simulink library "Rotation"  (R2018b)
settings: Solver=VariableStepAuto  StartTime=0.0  StopTime=10.0  RelTol=1e-3
settings Model: Creator=zouji  LastModifiedBy=zouji

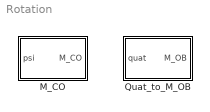
== system Rotation ==
  M_CO : Subsystem
  Quat_to_M_OB : Subsystem

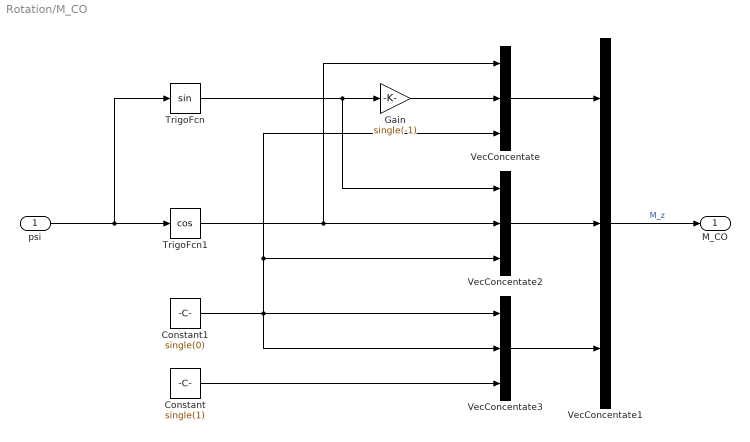
== system Rotation/M_CO ==
  psi : Inport  Unit=rad  PortDimensions=1
      settings: AttributesFormatString=Unit: %<Unit>
  Constant : Constant  Value=single(1)  VectorParams1D=off  OutDataTypeStr=Inherit: Inherit via back propagation
      settings: AttributesFormatString=Value: %<Value>
  Constant1 : Constant  Value=single(0)  VectorParams1D=off  OutDataTypeStr=Inherit: Inherit via back propagation
      settings: AttributesFormatString=Value: %<Value>
  Gain : Gain  Gain=single(-1)  OutDataTypeStr=Inherit: Same as input  ParamDataTypeStr=Inherit: Same as input
      settings: AttributesFormatString=Gain: %<Gain>
  TrigoFcn : Trigonometry  OutputSignalType=real
  TrigoFcn1 : Trigonometry  Operator=cos  OutputSignalType=real
  VecConcentate : Concatenate  NumInputs=3  Mode=Multidimensional array
  VecConcentate1 : Concatenate  NumInputs=3  Mode=Multidimensional array  ConcatenateDimension=2
  VecConcentate2 : Concatenate  NumInputs=3  Mode=Multidimensional array
  VecConcentate3 : Concatenate  NumInputs=3  Mode=Multidimensional array
  M_CO : Outport  Unit=1  PortDimensions=[3,3]
      settings: AttributesFormatString=Unit: %<Unit>
  wires:
  Constant1/1 -> VecConcentate/3, VecConcentate2/3, VecConcentate3/2, VecConcentate3/1
  TrigoFcn1/1 -> VecConcentate/1, VecConcentate2/2
  psi/1 -> TrigoFcn/1, TrigoFcn1/1
  VecConcentate1/1 -> M_CO/1  "M_z"
  VecConcentate/1 -> VecConcentate1/1
  VecConcentate2/1 -> VecConcentate1/2
  VecConcentate3/1 -> VecConcentate1/3
  TrigoFcn/1 -> VecConcentate2/1, Gain/1
  Gain/1 -> VecConcentate/2
  Constant/1 -> VecConcentate3/3

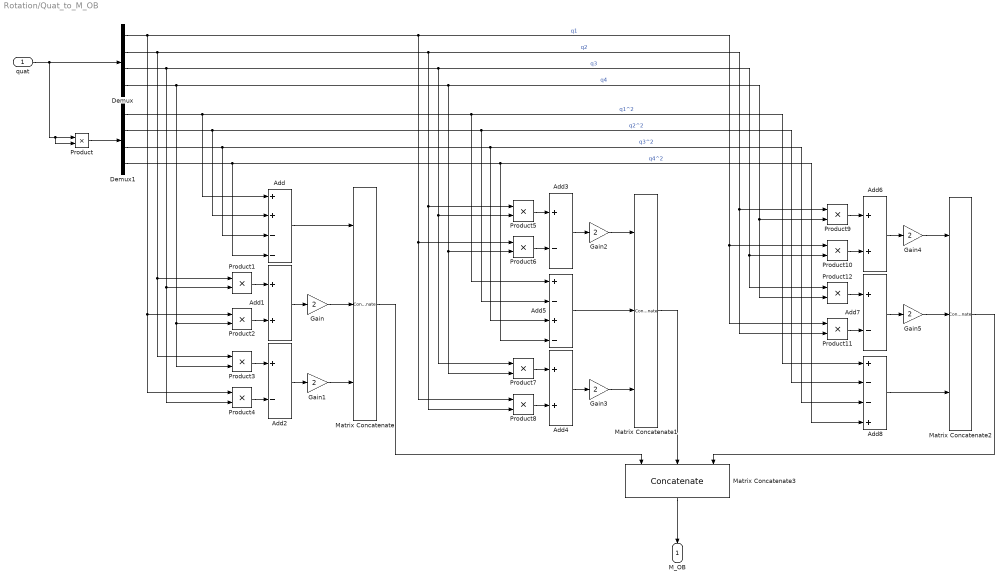
== system Rotation/Quat_to_M_OB ==
  quat : Inport
  Add : Sum  Inputs=++--
  Add1 : Sum
  Add2 : Sum  Inputs=+-
  Add3 : Sum  Inputs=+-
  Add4 : Sum
  Add5 : Sum  Inputs=+-+-
  Add6 : Sum
  Add7 : Sum  Inputs=+-
  Add8 : Sum  Inputs=+--+
  Demux : Demux
  Demux1 : Demux
  Gain{,1..5} (6 alike) : Gain  Gain=2  OutDataTypeStr=Inherit: Same as input
  Matrix Concatenate : Concatenate  NumInputs=3
  Matrix Concatenate1 : Concatenate  NumInputs=3
  Matrix Concatenate2 : Concatenate  NumInputs=3
  Matrix Concatenate3 : Concatenate  NumInputs=3  Mode=Multidimensional array  ConcatenateDimension=2
  Product{,1..12} (13 alike) : Product  RndMeth=Zero
  M_OB : Outport
  wires:
  Matrix Concatenate3/1 -> M_OB/1
  Matrix Concatenate2/1 -> Matrix Concatenate3/3
  Matrix Concatenate1/1 -> Matrix Concatenate3/2
  Matrix Concatenate/1 -> Matrix Concatenate3/1
  Add8/1 -> Matrix Concatenate2/3
  Gain5/1 -> Matrix Concatenate2/2
  Product11/1 -> Add7/2
  Product12/1 -> Add7/1
  Add7/1 -> Gain5/1
  Product10/1 -> Add6/2
  Product9/1 -> Add6/1
  Gain4/1 -> Matrix Concatenate2/1
  Add6/1 -> Gain4/1
  Add5/1 -> Matrix Concatenate1/2
  Gain3/1 -> Matrix Concatenate1/3
  Product8/1 -> Add4/2
  Product7/1 -> Add4/1
  Add4/1 -> Gain3/1
  Product6/1 -> Add3/2
  Product5/1 -> Add3/1
  Gain2/1 -> Matrix Concatenate1/1
  Add3/1 -> Gain2/1
  Gain1/1 -> Matrix Concatenate/3
  Product4/1 -> Add2/2
  Product3/1 -> Add2/1
  Add2/1 -> Gain1/1
  Product2/1 -> Add1/2
  Product1/1 -> Add1/1
  Gain/1 -> Matrix Concatenate/2
  Add1/1 -> Gain/1
  Add/1 -> Matrix Concatenate/1
  Demux/1 -> Product10/1, Product11/1, Product6/1, Product8/1, Product4/1, Product2/1  "q1"
  Demux/2 -> Product9/1, Product11/2, Product5/1, Product8/2, Product3/1, Product1/1  "q2"
  Demux/3 -> Product5/2, Product7/1, Product12/1, Product10/2, Product4/2, Product1/2  "q3"
  Demux/4 -> Product9/2, Product12/2, Product6/2, Product7/2, Product3/2, Product2/2  "q4"
  Demux1/4 -> Add8/4, Add5/4, Add/4  "q4^2"
  Demux1/3 -> Add8/3, Add5/3, Add/3  "q3^2"
  Demux1/2 -> Add8/2, Add5/2, Add/2  "q2^2"
  Demux1/1 -> Add8/1, Add5/1, Add/1  "q1^2"
  Product/1 -> Demux1/1
  quat/1 -> Demux/1, Product/2, Product/1
